simulink model "aero_bf"  (R2013a)
settings: Solver=ode5  SolverMode=SingleTasking  StartTime=0.0  StopTime=inf  FixedStep=Ts  RelTol=1e-3
values from neighbouring files (symbols this model uses):
  R = [r10 r11 r12]    [Aero_init.m]
  S = [1 (sp11-1) -sp11]    [Aero_init.m]
  T = r10+ r11+ r12    [Aero_init.m]
  Te = 2.0    (= 2)    [Aero_init.m]
  Ts = 0.1    [Aero_init.m]
  U0 = 5    [Aero_init.m]
  V0 = 6    [Aero_init.m]
undefined symbols (not defined in the file or in its folder): Standard_Devices, UDP_Protocol
libraries: etargetslib x13, rtwinlib x2, simulink_extras x2, simulink x1
CloseFcn:
  | rtwprivate ssgencode ModelCloseRequest aero_bf
settings Model: SimulationMode=external  ExtModeTrigDuration=6000  Creator=drey  LastModifiedBy=adm.e3.bucheg
settings DataIOCC: LimitDataPoints=off  SignalLoggingSaveFormat=ModelDataLogs
settings OptimizationCC: BlockReduction=off  BooleanDataType=off  ExpressionDepthLimit=2147483647  InitFltsAndDblsToZero=on
settings DebuggingCC: SaveWithParameterizedLinksMsg=none  SignalResolutionControl=TryResolveAllWithWarning  SolverPrmCheckMsg=none  MultiTaskDSMMsg=warning  MultiTaskCondExecSysMsg=none  FcnCallInpInsideContextMsg=UseLocalSettings  StrictBusMsg=None
settings RTWCC: SystemTargetFile=rtwin.tlc  TemplateMakefile=rtwin.tmf  Description=Real-Time Windows Target  RTWVerbose=off  ProcessScript=rtwin_make_rtw_hook  IncludeERTFirstTime=on
settings RTWinTargetCC: TargetFcnLib=ansi_tfl_tmw.mat  TargetLibSuffix=_rtwin.lib  TargetPreCompLibLocation=C:\Program Files\MATLAB\R2013a\toolbox\rtw\targets\rtwin\lib\win64  CodeReplacementLibrary=ANSI_C  ModelReferenceCompliant=off  CompOptLevelCompliant=off  RTWinDir=C:/PROGRA~1/MATLAB/R2013a/toolbox/rtw/targets/rtwin  TargetArch=win64

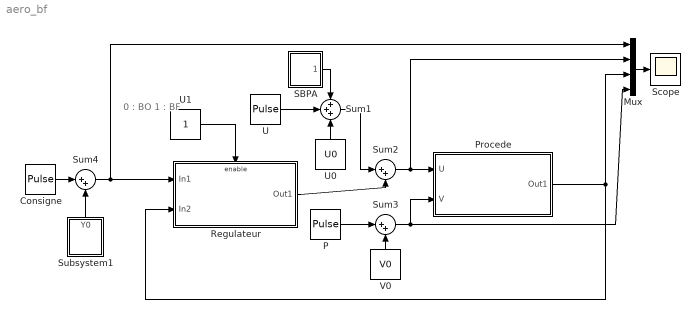
== system aero_bf ==
  note: 0 : BO
      | 1 : BF
  Consigne : DiscretePulseGenerator  PulseType=Time based  Amplitude=0.5  Period=200  PulseWidth=50  PhaseDelay=100
  Mux : Mux
  P : DiscretePulseGenerator  PulseType=Time based  Amplitude=0  Period=200  PulseWidth=50  PhaseDelay=100
  Procede : Subsystem
      mask Display: disp('Procede')
  Regulateur : Subsystem  TreatAsAtomicUnit=on
      mask Display: disp('Regulateur')
  SBPA : Subsystem  mask(Configuration d'une SBPA){Nfr=4, Ifr=[1 0 1 0], Nsr=3, Isr=[1 0 1], A=0, Te=2*Te}
      mask prompts: Nfr "The first register length"; Ifr "Initialisation of the first reg"; Nsr "The second register length"; Isr "Initialisation of the sec reg"; A "Amplitude"; Te "Sample Time"
      mask help:
      | Note Importante:
      | Le choix du degré du registre principal et du sample time est déterminé par le temps de montée du procédé. La relation a respecter est :
      |                                         tm >= L * Ts
      | L = nbr de zéros dans les denom et num du registre
      | Ts = Sample Time
      | Pour plus de renseignements voir l'aide
      mask Help:
      | Cette SBPA est construite à l'aide de bloc discret en Z représentant des registres binaires.
      | L'aspect aléatoire des valeurs est obtenu par un modulo 2 entre certains bits de ce registre.
      | Il s'agit donc ici de déterminer la taille de ces registres qui correspondent en fait aux degrés des blocs discrets.
      | Exemple de configuration suivant les champs
      | 1)=: [1 0 0 0]                   //
      | 2)=: [0 0 0 1]                   // Reg modulo = 1/Z^3
      | 3)=: [1 0 1]                      // Init du reg
      | 4)=: [1 0 1 0 1 0 1 0]     // Init du reg principal
      | 5)=: [1 0 0 0 0 0 0]        //
      | 6)=: [0 0 0 0 0 0 1]        // Reg principal = 1/Z^6
      mask Display: disp('Sbpa')
  Scope : Scope
      settings: TimeRange=600  YMin=3.5  YMax=6.5  SaveName=X  MaxDataPoints=80000
  Subsystem1 : Subsystem
      mask Display: disp('Y0')
  Sum1 : Sum  Inputs=+++  SaturateOnIntegerOverflow=on  InputSameDT=on  OutDataTypeStr=Inherit: Same as first input
  Sum2 : Sum  Inputs=|++  SaturateOnIntegerOverflow=on  InputSameDT=on  OutDataTypeStr=Inherit: Same as first input
  Sum3 : Sum  Inputs=|++  SaturateOnIntegerOverflow=on  InputSameDT=on  OutDataTypeStr=Inherit: Same as first input
  Sum4 : Sum  Inputs=|++  SaturateOnIntegerOverflow=on  InputSameDT=on  OutDataTypeStr=Inherit: Same as first input
  U : DiscretePulseGenerator  PulseType=Time based  Amplitude=0  Period=200  PulseWidth=50  PhaseDelay=20
  U0 : Constant  Value=U0
  U1 : Constant
  V0 : Constant  Value=V0
  wires:
  Regulateur/1(Out1) -> Sum2/2
  Sum2/1 -> Procede/1(U), Mux/2
  Sum1/1 -> Sum2/1
  Mux/1 -> Scope/1
  P/1 -> Sum3/1
  V0/1 -> Sum3/2
  Sum3/1 -> Mux/4, Procede/2(V)
  Procede/1(Out1) -> Mux/3, Regulateur/2(In2)
  Sum4/1 -> Mux/1, Regulateur/1(In1)
  Consigne/1 -> Sum4/1
  Subsystem1/1(Y0) -> Sum4/2
  U1/1 -> Regulateur/Enable
  U/1 -> Sum1/2
  U0/1 -> Sum1/3
  SBPA/1(Out1) -> Sum1/1

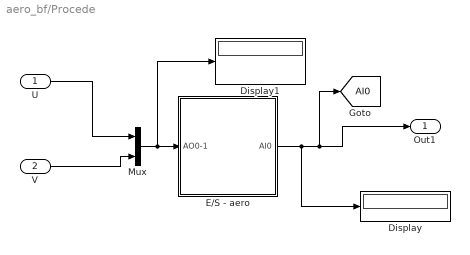
== system aero_bf/Procede ==
  U : Inport
  V : Inport  Port=2
  Display : Display
  Display1 : Display
  E/S - aero : Subsystem
  Mux : Mux  Inputs=2
  Out1 : Outport
  tag scope: AI0=global
  wires:
  Mux/1 -> Display1/1, E/S - aero/1("AO0-1 ")
  U/1 -> Mux/1
  V/1 -> Mux/2
  E/S - aero/1(AI0) -> Display/1, [AI0], Out1/1

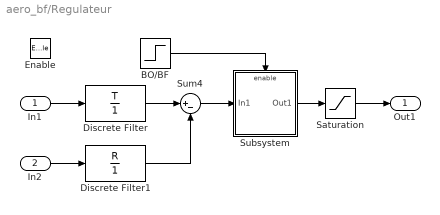
== system aero_bf/Regulateur ==
  In1 : Inport
  In2 : Inport  Port=2
  Enable : EnablePort
  BO/BF : Step  Time=10  SampleTime=Ts
  Discrete Filter : DiscreteFilter  Numerator=T  Denominator=1  SampleTime=Te
  Discrete Filter1 : DiscreteFilter  Numerator=R  Denominator=1  SampleTime=Te
  Saturation : Saturate  UpperLimit=10-U0  LowerLimit=0-U0
  Subsystem : Subsystem  TreatAsAtomicUnit=on
      mask Display: disp('1/S(z)')
  Sum4 : Sum  Inputs=|+-  SaturateOnIntegerOverflow=on  InputSameDT=on  OutDataTypeStr=Inherit: Same as first input
  Out1 : Outport
  wires:
  Sum4/1 -> Subsystem/1(In1)
  Discrete Filter/1 -> Sum4/1
  In1/1 -> Discrete Filter/1
  Subsystem/1(Out1) -> Saturation/1
  Saturation/1 -> Out1/1
  In2/1 -> Discrete Filter1/1
  Discrete Filter1/1 -> Sum4/2
  BO/BF/1 -> Subsystem/Enable

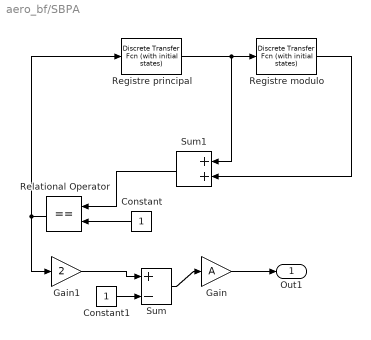
== system aero_bf/SBPA ==
  Constant : Constant
  Constant1 : Constant
  Gain : Gain  Gain=A  SaturateOnIntegerOverflow=on  OutDataTypeStr=Inherit: Same as input  ParamDataTypeStr=Inherit: Same as input
  Gain1 : Gain  Gain=2  SaturateOnIntegerOverflow=on  OutDataTypeStr=Inherit: Same as input  ParamDataTypeStr=Inherit: Same as input
  Registre modulo : simulink_extras/Additional Discrete/Discrete Transfer Fcn (with initial states)  N=[zeros(1,Nsr) 1]  D=[1 zeros(1,Nsr)]  X0=Isr  TS=Te
  Registre principal : simulink_extras/Additional Discrete/Discrete Transfer Fcn (with initial states)  N=[zeros(1,Nfr) 1]  D=[1 zeros(1,Nfr)]  X0=Ifr  TS=Te
  Relational Operator : RelationalOperator  Operator===  InputSameDT=on
  Sum : Sum  Inputs=|+-  SaturateOnIntegerOverflow=on  InputSameDT=on  OutDataTypeStr=Inherit: Same as first input
  Sum1 : Sum  SaturateOnIntegerOverflow=on  InputSameDT=on  OutDataTypeStr=Inherit: Same as first input
  Out1 : Outport
  wires:
  Sum1/1 -> Relational Operator/1
  Registre modulo/1 -> Sum1/2
  Constant/1 -> Relational Operator/2
  Registre principal/1 -> Sum1/1, Registre modulo/1
  Relational Operator/1 -> Registre principal/1, Gain1/1
  Gain1/1 -> Sum/1
  Constant1/1 -> Sum/2
  Sum/1 -> Gain/1
  Gain/1 -> Out1/1

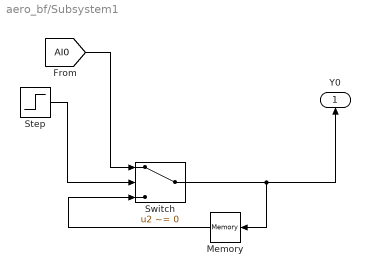
== system aero_bf/Subsystem1 ==
  Memory : Memory
  Step : Step  Before=1  After=0  SampleTime=Ts
  Switch : Switch  Criteria=u2 ~= 0
  Y0 : Outport
  wires:
  [AI0] -> Switch/1
  Switch/1 -> Memory/1, Y0/1
  Memory/1 -> Switch/3
  Step/1 -> Switch/2

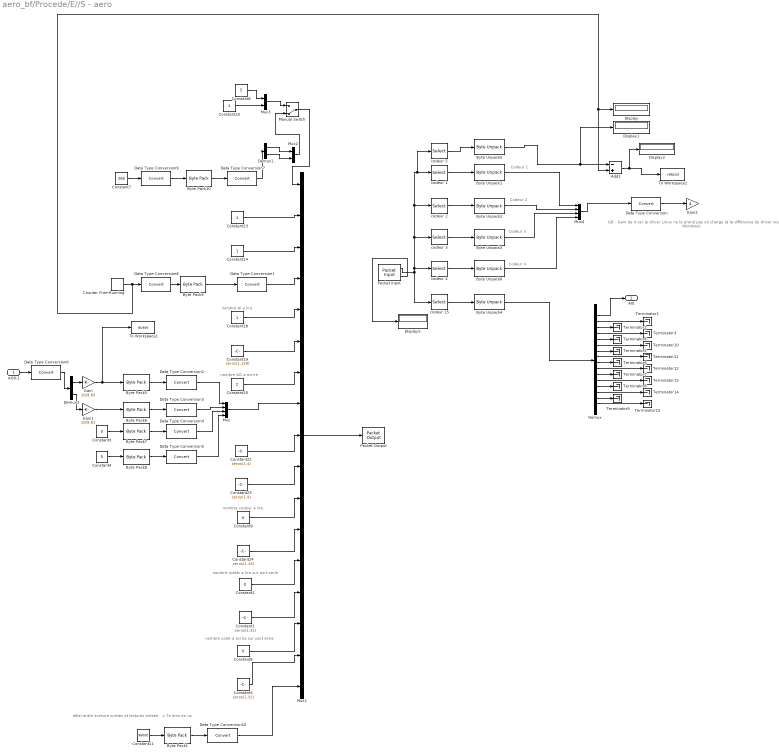
== system aero_bf/Procede/E//S - aero ==
  note: delai entre ecriture sorties et lectures entrée : = Ts-4ms en us
  note: Codeur 4
  note: Codeur 3
  note: Codeur 2
  note: Codeur 1
  note: GB : Gain de 4 car le driver Linux
      |  ne le prend pas en charge
      | (à la différence du driver sous Windows)
  note: nombre AO a ecrire
  note: nombre AI a lire
  note: nombre codeur a lire
  note: nombre octets a lire sur port serie
  note: nombre octet a ecrire sur port serie
  "AO0-1 " : Inport
  Add1 : Sum  Inputs=-+
  Byte Pack1 : etargetslib/Byte Pack  datatypes={'uint32'}  byteAlign=1
  Byte Pack10 : etargetslib/Byte Pack  datatypes={'int16'}  byteAlign=1
  Byte Pack{5..8} (4 alike) : etargetslib/Byte Pack  datatypes={'double'}  byteAlign=1
  Byte Pack9 : etargetslib/Byte Pack  datatypes={'uint32'}  byteAlign=1
  Byte Unpack{1..3,6} (4 alike) : etargetslib/Byte Unpack  dimensions={[1]}  datatypes={'int32'}  byteAlign=4
  Byte Unpack4 : etargetslib/Byte Unpack  dimensions={[16]}  datatypes={'double'}  byteAlign=4
  Byte Unpack5 : etargetslib/Byte Unpack  dimensions={[1]}  datatypes={'uint32'}  byteAlign=4
  Constant1 : Constant  Value=zeros(1,32)
  Constant{10,13..14,18} (4 alike) : Constant
  Constant11 : Constant  Value=96000  OutDataTypeStr=uint32
  Constant19 : Constant  Value=zeros(1,128)
  Constant2 : Constant  Value=0
  Constant20 : Constant  Value=2  OutDataTypeStr=Inherit: Inherit via back propagation
  Constant22 : Constant  Value=zeros(1,4)
  Constant23 : Constant  Value=zeros(1,4)
  Constant24 : Constant  Value=zeros(1,16)
  Constant3 : Constant  Value=0  OutDataTypeStr=double
  Constant4 : Constant  Value=0  OutDataTypeStr=double
  Constant5 : Constant  Value=zeros(1,32)
  Constant6 : Constant  Value=0
  Constant7 : Constant  Value=265
  Constant8 : Constant  Value=5
  Constant9 : Constant  Value=0
  Counter Free-Running : simulink/Sources/Counter Free-Running  NumBits=32  tsamp=-1
  Data Type Conversion{,1..10} (11 alike) : DataTypeConversion
  Demux : Demux  Outputs=16
  Demux1 : Demux  Outputs=2
  Demux2 : Demux  Outputs=2
  Display{,1..2,5} (4 alike) : Display
  Gain : Gain  Gain=10/9.83
  Gain1 : Gain  Gain=10/9.81
  Gain2 : Gain  Gain=4
  Manual Switch : ManualSwitch  CurrentSetting=0
  Mux : Mux
  Mux1 : Mux  Inputs=17
  Mux2 : Mux  Inputs=2
  Mux3 : Mux  Inputs=2
  Mux4 : Mux
  Packet Input : rtwinlib/Packet Input  SampleTime=Ts  MaxMissedTicks=10  ShowMissedTicks=on  YieldWhenWaiting=off  DrvName=Standard_Devices/UDP_Protocol  DrvAddress=9930  DrvOptions=[3232235522 9930]  PacketSize=265  DataTypes='265*uint8'  ShowReady=off  ShowError=off  PacketID=1  ByteOrder=1  ShowTimestamp=off
      settings: AttributesFormatString=Standard Devices\nUDP Protocol [26CAh]
  Packet Output : rtwinlib/Packet Output  SampleTime=Ts  MaxMissedTicks=10  ShowMissedTicks=off  YieldWhenWaiting=off  DrvName=Standard_Devices/UDP_Protocol  DrvAddress=9930  DrvOptions=[3232235522 9930]  PacketSize=265  DataTypes='265*uint8'  ShowReady=off  ShowError=off  PacketID=1  ByteOrder=1  InitialValue=[]  FinalValue=[]
      settings: AttributesFormatString=Standard Devices\nUDP Protocol [26CAh]
  Terminator{1..15} (15 alike) : Terminator
  To Workspace1 : ToWorkspace  VariableName=aoser  SampleTime=-1  SaveFormat=Structure With Time
  To Workspace2 : ToWorkspace  VariableName=retard  SampleTime=-1  SaveFormat=Structure With Time
  codeur 1 : Selector  InputPortWidth=265  IndexOptions=Index vector (dialog)  Indices=[180 181 182 183]  OutputSizes=1
  codeur 15 : Selector  InputPortWidth=265  IndexOptions=Index vector (dialog)  Indices=[10:137]  OutputSizes=1
  codeur 2 : Selector  InputPortWidth=265  IndexOptions=Index vector (dialog)  Indices=[184 185 186 187]  OutputSizes=1
  codeur 3 : Selector  InputPortWidth=265  IndexOptions=Index vector (dialog)  Indices=[188 189 190 191]  OutputSizes=1
  codeur 4 : Selector  InputPortWidth=265  IndexOptions=Index vector (dialog)  Indices=[192 193 194 195]  OutputSizes=1
  codeur 5 : Selector  InputPortWidth=265  IndexOptions=Index vector (dialog)  Indices=[5 6 7 8]  OutputSizes=1
  AI0 : Outport
  wires:
  Constant13/1 -> Mux1/2
  Constant14/1 -> Mux1/3
  Constant18/1 -> Mux1/5
  Constant19/1 -> Mux1/6
  Constant20/1 -> Mux1/7
  Mux/1 -> Mux1/8
  Constant22/1 -> Mux1/9
  Constant23/1 -> Mux1/10
  Constant9/1 -> Mux1/11
  Constant24/1 -> Mux1/12
  Mux1/1 -> Packet Output/1
  Data Type Conversion5/1 -> Mux/4
  Data Type Conversion4/1 -> Mux/3
  Constant3/1 -> Byte Pack7/1
  Constant4/1 -> Byte Pack8/1
  Data Type Conversion1/1 -> Mux1/4
  Byte Pack8/1 -> Data Type Conversion5/1
  Byte Pack7/1 -> Data Type Conversion4/1
  Data Type Conversion2/1 -> Mux/1
  Byte Pack5/1 -> Data Type Conversion2/1
  Data Type Conversion3/1 -> Mux/2
  Byte Pack6/1 -> Data Type Conversion3/1
  codeur 15/1 -> Byte Unpack4/1
  Constant1/1 -> Mux1/14
  Constant2/1 -> Mux1/13
  Constant6/1 -> Mux1/15
  Constant7/1 -> Data Type Conversion9/1
  Byte Pack10/1 -> Data Type Conversion7/1
  Packet Input/1 -> codeur 15/1, codeur 5/1, codeur 1/1, codeur 2/1, codeur 3/1, codeur 4/1
  Data Type Conversion7/1 -> Demux1/1
  Manual Switch/1 -> Mux1/1
  Mux3/1 -> Manual Switch/1
  Constant10/1 -> Mux3/2
  Constant8/1 -> Mux3/1
  Mux4/1 -> Data Type Conversion/1
  "AO0-1 "/1 -> Data Type Conversion6/1
  Constant5/1 -> Mux1/16
  Data Type Conversion/1 -> Gain2/1
  Data Type Conversion6/1 -> Demux2/1
  Data Type Conversion8/1 -> Byte Pack9/1
  Demux2/2 -> Gain1/1
  Demux2/1 -> Gain/1
  Gain/1 -> To Workspace1/1, Byte Pack5/1
  Gain1/1 -> Byte Pack6/1
  Mux2/1 -> Manual Switch/2
  Data Type Conversion9/1 -> Byte Pack10/1
  codeur 1/1 -> Byte Unpack1/1
  Byte Unpack1/1 -> Mux4/1
  codeur 2/1 -> Byte Unpack2/1
  codeur 3/1 -> Byte Unpack3/1
  codeur 4/1 -> Byte Unpack6/1
  Byte Unpack6/1 -> Mux4/4
  Byte Unpack3/1 -> Mux4/3
  Byte Unpack2/1 -> Mux4/2
  Byte Unpack4/1 -> Demux/1
  Demux/2 -> Terminator1/1
  Demux/3 -> Terminator2/1
  Demux/4 -> Terminator3/1
  Demux/8 -> Terminator11/1
  Demux/6 -> Terminator10/1
  Demux/5 -> Terminator4/1
  Demux/9 -> Terminator6/1
  Demux/7 -> Terminator5/1
  Demux/10 -> Terminator12/1
  Demux/11 -> Terminator7/1
  Demux/13 -> Terminator8/1
  Demux/15 -> Terminator9/1
  Demux/12 -> Terminator13/1
  Demux/14 -> Terminator14/1
  Demux/16 -> Terminator15/1
  codeur 5/1 -> Byte Unpack5/1
  Byte Unpack5/1 -> Display1/1, Add1/1
  Byte Pack9/1 -> Data Type Conversion1/1
  Counter Free-Running/1 -> Add1/2, Display/1, Data Type Conversion8/1
  Constant11/1 -> Byte Pack1/1
  Byte Pack1/1 -> Data Type Conversion10/1
  Data Type Conversion10/1 -> Mux1/17
  Add1/1 -> Display2/1, To Workspace2/1
  Packet Input/2 -> Display5/1
  Demux1/2 -> Mux2/2
  Demux1/1 -> Mux2/1
  Demux/1 -> AI0/1

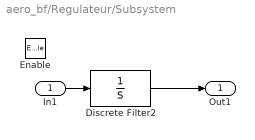
== system aero_bf/Regulateur/Subsystem ==
  In1 : Inport
  Enable : EnablePort
  Discrete Filter2 : DiscreteFilter  Numerator=1  Denominator=S  SampleTime=Te
  Out1 : Outport
  wires:
  In1/1 -> Discrete Filter2/1
  Discrete Filter2/1 -> Out1/1
